simulink model "proiect_P1_R2024b"  (R2024b)
settings: Solver=FixedStepAuto  StartTime=0.0  StopTime=Tfin  FixedStep=Ts  RelTol=1e-3
values from neighbouring files (symbols this model uses):
  a0 = (1000+n*200)^2    (= 3240000)    [proiect_P1_setup.m]
  a1 = 2*(0.2+m/20)*(1000+n*200)    (= 720)    [proiect_P1_setup.m]
  b0 = (2.2+m+n)*(1000+n*200)^2    (= 20088000)    [proiect_P1_setup.m]
  t1 = 10/a1    (= 0.0138888888889)    [proiect_P1_setup.m]
  Ts = 20/a1/1e4    (= 2.77777777778e-06)    [proiect_P1_setup.m]
  u0 = 0    [proiect_P1_setup.m]
  umax = 15    [proiect_P1_setup.m]
  umin = -15    [proiect_P1_setup.m]
  ust = 1    [proiect_P1_setup.m]
  whtn_pow_in = 1e-7/2    (= 5e-08)    [proiect_P1_setup.m]
  whtn_pow_out = 1e-6/2    (= 5e-07)    [proiect_P1_setup.m]
  whtn_seed_in = 23341    [proiect_P1_setup.m]
  whtn_seed_out = 23342    [proiect_P1_setup.m]
  whtn_Ts_in = Ts    (= 2.77777777778e-06)    [proiect_P1_setup.m]
  whtn_Ts_out = Ts*5    (= 1.38888888889e-05)    [proiect_P1_setup.m]
  x0 = [-1e-5*m; (-1)^m*1e-7*2*n]    [proiect_P1_setup.m]
  ymax = 24    [proiect_P1_setup.m]
  ymin = -24    [proiect_P1_setup.m]
libraries: simulink x4
settings Model: Creator=mircea  LastModifiedBy=vladmihaly

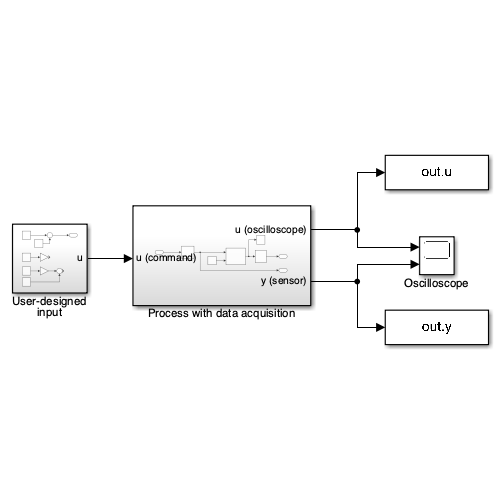
[thumbnail: Simulink's stored preview of the top-level diagram]
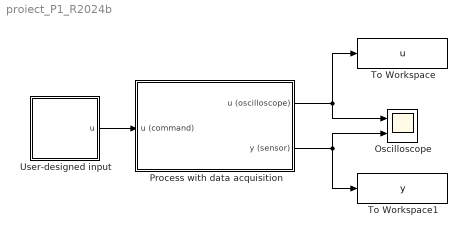
== system proiect_P1_R2024b ==
  Oscilloscope : Scope  NumInputPorts=2
  Process with data acquisition : Subsystem
  To Workspace : ToWorkspace  VariableName=u  SampleTime=Ts
  To Workspace1 : ToWorkspace  VariableName=y  SampleTime=Ts
  User-designed input : Subsystem
  wires:
  Process with data acquisition/1(u (oscilloscope)) -> Oscilloscope/1, To Workspace/1
  Process with data acquisition/2(y (sensor)) -> Oscilloscope/2, To Workspace1/1
  User-designed input/1(u) -> Process with data acquisition/1(u (command))

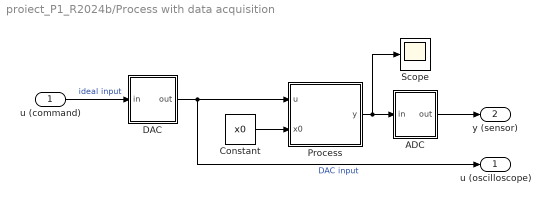
== system proiect_P1_R2024b/Process with data acquisition ==
  u (command) : Inport
  ADC : Subsystem
  Constant : Constant  Value=x0
  DAC : Subsystem
  Process : Subsystem
  Scope : Scope
  u (oscilloscope) : Outport
  y (sensor) : Outport  Port=2
  wires:
  Constant/1 -> Process/2(x0)
  u (command)/1 -> DAC/1(in)  "ideal input"
  Process/1(y) -> Scope/1, ADC/1(in)
  ADC/1(out) -> y (sensor)/1
  DAC/1(out) -> Process/1(u), u (oscilloscope)/1  "DAC input"

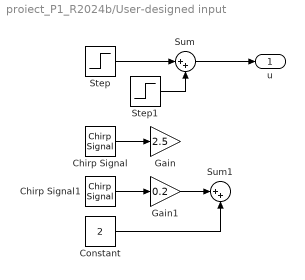
== system proiect_P1_R2024b/User-designed input ==
  Chirp Signal : simulink/Sources/Chirp Signal  f1=0.01  T=80  f2=15
  Chirp Signal1 : simulink/Sources/Chirp Signal  f1=0.01  T=80  f2=15
  Constant : Constant  Value=2
  Gain : Gain  Gain=2.5
  Gain1 : Gain  Gain=0.2
  Step : Step  Time=t1  Before=u0  After=ust  SampleTime=0
  Step1 : Step  Time=2*t1  Before=u0  After=ust  SampleTime=0
  Sum : Sum  Inputs=|++
  Sum1 : Sum  Inputs=|++
  u : Outport
  wires:
  Chirp Signal/1 -> Gain/1
  Step/1 -> Sum/1
  Step1/1 -> Sum/2
  Chirp Signal1/1 -> Gain1/1
  Gain1/1 -> Sum1/1
  Constant/1 -> Sum1/2
  Sum/1 -> u/1

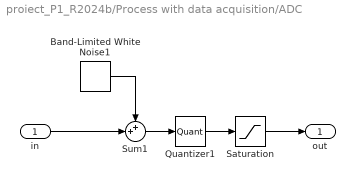
== system proiect_P1_R2024b/Process with data acquisition/ADC ==
  in : Inport
  Band-Limited White Noise1 : simulink/Sources/Band-Limited White Noise  Cov=[whtn_pow_out]  Ts=whtn_Ts_out  seed=[whtn_seed_out]
  Quantizer1 : Quantizer  QuantizationInterval=q_out
  Saturation : Saturate  UpperLimit=ymax  LowerLimit=ymin
  Sum1 : Sum  Inputs=++|
  out : Outport
  wires:
  Quantizer1/1 -> Saturation/1
  Sum1/1 -> Quantizer1/1
  in/1 -> Sum1/2
  Band-Limited White Noise1/1 -> Sum1/1
  Saturation/1 -> out/1

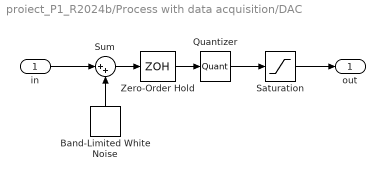
== system proiect_P1_R2024b/Process with data acquisition/DAC ==
  in : Inport
  Band-Limited White Noise : simulink/Sources/Band-Limited White Noise  Cov=[whtn_pow_in]  Ts=whtn_Ts_in  seed=[whtn_seed_in]
  Quantizer : Quantizer  QuantizationInterval=q_in
  Saturation : Saturate  UpperLimit=umax  LowerLimit=umin
  Sum : Sum  Inputs=|++
  Zero-Order Hold : ZeroOrderHold  SampleTime=-1
  out : Outport
  wires:
  Quantizer/1 -> Saturation/1
  Sum/1 -> Zero-Order Hold/1
  in/1 -> Sum/1
  Band-Limited White Noise/1 -> Sum/2
  Zero-Order Hold/1 -> Quantizer/1
  Saturation/1 -> out/1

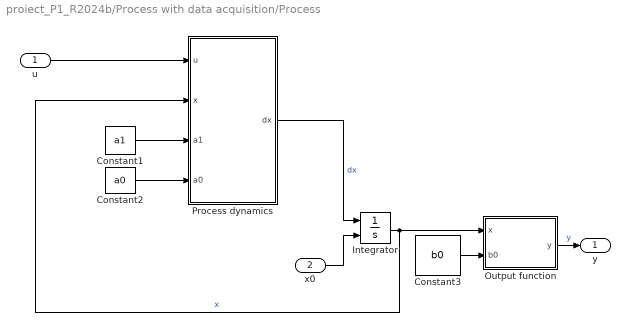
== system proiect_P1_R2024b/Process with data acquisition/Process ==
  u : Inport
  x0 : Inport  Port=2
  Constant1 : Constant  Value=a1
  Constant2 : Constant  Value=a0
  Constant3 : Constant  Value=b0
  Integrator : Integrator  InitialConditionSource=external
  Output function : MATLAB Function  TreatAsAtomicUnit=on
  Process dynamics : MATLAB Function  TreatAsAtomicUnit=on
  y : Outport
  wires:
  u/1 -> Process dynamics/1(u)
  Process dynamics/1(dx) -> Integrator/1  "dx"
  Integrator/1 -> Output function/1(x), Process dynamics/2(x)  "x"
  Output function/1(y) -> y/1  "y"
  x0/1 -> Integrator/2
  Constant2/1 -> Process dynamics/4(a0)
  Constant1/1 -> Process dynamics/3(a1)
  Constant3/1 -> Output function/2(b0)

== matlab function proiect_P1_R2024b/Process with data acquisition/Process/Process dynamics ==
  data: u input; dx output; x input; a1 input; a0 input
function dx = fcn(u,x,a1,a0)
dx = [-a1*x(1) - a0*x(2)+u; x(1)];

== matlab function proiect_P1_R2024b/Process with data acquisition/Process/Output function ==
  data: y output; x input; b0 input
function y = fcn(x,b0)

y = b0*x(2);

end
